simulink model "taskKoshi"  (Simulink 7.9)
settings: Solver=ode45  StartTime=-10.0  StopTime=10.0  RelTol=1e-3
libraries: simulink x2
settings Model: Creator=Mihail  LastModifiedBy=Mihail

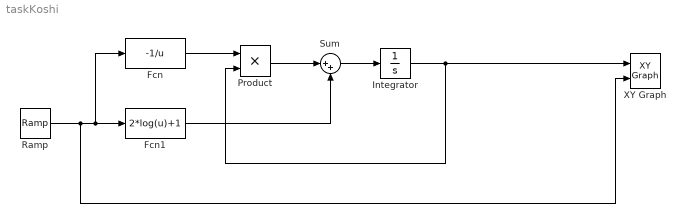
== system taskKoshi ==
  Fcn : Fcn  Expr=-1/u
  Fcn1 : Fcn  Expr=2*log(u)+1
  Integrator : Integrator  InitialCondition=1
  Product : Product  RndMeth=Zero
  Ramp : simulink/Sources/Ramp  slope=1  start=1  X0=1
  Sum : Sum  Inputs=|++
  XY Graph : simulink/Sinks/XY Graph  xmin=-5  xmax=5  ymin=-5  ymax=5  st=-1
  wires:
  Ramp/1 -> XY Graph/2, Fcn1/1, Fcn/1
  Integrator/1 -> Product/2, XY Graph/1
  Product/1 -> Sum/1
  Sum/1 -> Integrator/1
  Fcn/1 -> Product/1
  Fcn1/1 -> Sum/2
